simulink model "ADRC_main"  (R2015a)
settings: Solver=ode1  StartTime=0.0  StopTime=100  FixedStep=0.01  RelTol=1e-3
model workspace (MATLAB code in the model file):
  | r=10;T=0.01;h=0.1;bet=[1/h 1/(1.6*h^1.5) 1/(8.6*h^2.2)];d=h;b=1;aa=[0.75 1.25];bet1=[100 10];
settings Model: Creator=lenovo  LastModifiedBy=lenovo

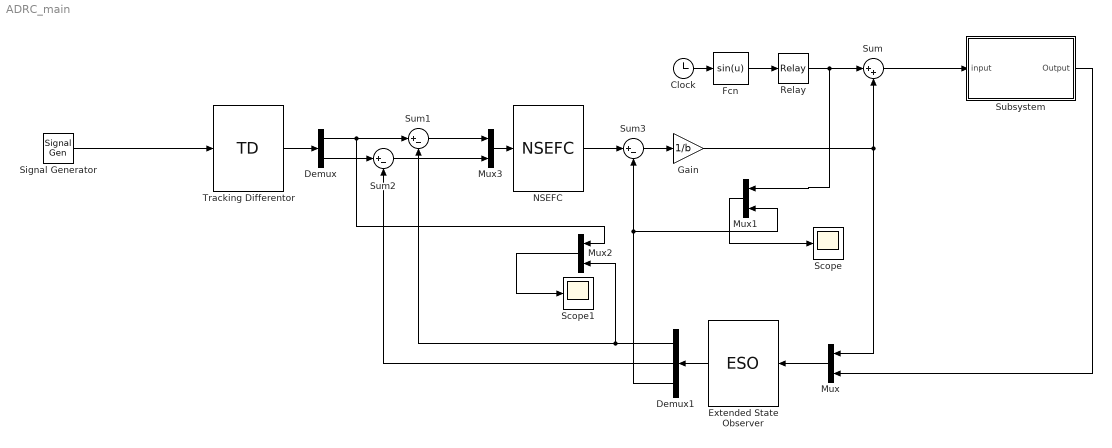
== system ADRC_main ==
  Clock : Clock
  Demux : Demux  Outputs=2
  Demux1 : Demux  Outputs=3
  Extended State Observer : S-Function  FunctionName=ESO  Parameters=d,bet,b,T
  Fcn : Fcn  Expr=sin(u)
  Gain : Gain  Gain=1/b
  Mux{,1..3} (4 alike) : Mux  Inputs=2
  "NSEFC " : S-Function  FunctionName=NSEFC  Parameters=aa,bet1,d
  Relay : Relay
  Scope : Scope
  Scope1 : Scope
  Signal Generator : SignalGenerator  WaveForm=square  Frequency=0.1
  Subsystem : Subsystem
  Sum : Sum  Inputs=|++  SaturateOnIntegerOverflow=on  InputSameDT=on  OutDataTypeStr=Inherit: Same as first input
  Sum1 : Sum  Inputs=|+-
  Sum2 : Sum  Inputs=|+-
  Sum3 : Sum  Inputs=|+-
  Tracking Differentor : S-Function  FunctionName=TD  Parameters=r,h,T
  wires:
  Signal Generator/1 -> Tracking Differentor/1
  Tracking Differentor/1 -> Demux/1
  Extended State Observer/1 -> Demux1/1
  Mux/1 -> Extended State Observer/1
  Demux/2 -> Sum2/1
  Demux/1 -> Mux2/1, Sum1/1
  Sum1/1 -> Mux3/1
  Sum2/1 -> Mux3/2
  Demux1/1 -> Mux2/2, Sum1/2
  Demux1/2 -> Sum2/2
  Mux3/1 -> "NSEFC "/1
  Demux1/3 -> Mux1/2, Sum3/2
  "NSEFC "/1 -> Sum3/1
  Sum3/1 -> Gain/1
  Gain/1 -> Sum/2, Mux/1
  Subsystem/1(Output) -> Mux/2
  Clock/1 -> Fcn/1
  Fcn/1 -> Relay/1
  Relay/1 -> Mux1/1, Sum/1
  Sum/1 -> Subsystem/1(input)
  Mux1/1 -> Scope/1
  Mux2/1 -> Scope1/1

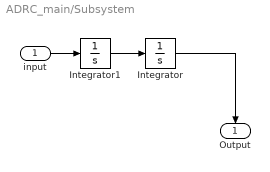
== system ADRC_main/Subsystem ==
  input : Inport
  Integrator : Integrator
  Integrator1 : Integrator
  Output : Outport
  wires:
  input/1 -> Integrator1/1
  Integrator1/1 -> Integrator/1
  Integrator/1 -> Output/1
